simulink model "Main_C0_C3"  (R2023a)
settings: Solver=ode15s  StartTime=0.0  StopTime=1  RelTol=1e-3
model workspace (MAT data in the model file):
  C_IVD = 0.05
  E_IVD1 = 2.1
  E_IVD2 = 2.2
  E_IVD3 = 1.1
  E_IVD4 = 1.7
  E_IVD5 = 3.2
  IVD1 : object (value not decoded)
  IVD2 : object (value not decoded)
  IVD3 : object (value not decoded)
  IVD4 : object (value not decoded)
  IVD5 : object (value not decoded)
  eo_color = [1 0 0]
  io_color = [0 1 0]
  longissimus_color = [1 0 1]
  multifidus_color = [0 1 1]
  muscle_radius = 1
  psoas_color = [0 0 1]
  ra_color = [1 1 0.5]
symbols that are objects in the model workspace (value not decoded): IVD1, IVD2, IVD3, IVD4, IVD5
undefined symbols (not defined in the file or in its folder): AbdFlex, E_TLFflex, IAP_activation_AbdFlex, IAP_Pa, LeftAbdominalMuscleForce, LeftBackMuscleForce, LeftTransverse1MuscleForce, LeftTransverse2MuscleForce, RightAbdominalMuscleForce, RightBackMuscleForce, RightTransverse1MuscleForce, RightTransverse2MuscleForce, TLFflex2, X, Y, Z
libraries: nesl_utility x1235, sm_lib x960, fl_lib x6, simulink_extras x2
(part 12 of 37)

== system Main_C0_C3/Left and Right Intertransverse Ligaments/ITL Visualization - debug/Ligament9 ==
  Constant : Constant  Value=0
  Constant1 : Constant  Value=0
  Gimbal Joint : sm_lib/Joints/Gimbal Joint  JointMode=Normal  SenseConstraintForce=off  SenseConstraintForceX=off  SenseConstraintForceY=off  SenseConstraintForceZ=off  SenseConstraintTorque=off  SenseConstraintTorqueX=off  SenseConstraintTorqueY=off  SenseConstraintTorqueZ=off  SenseTotalForce=off  SenseTotalForceX=off  SenseTotalForceY=off  SenseTotalForceZ=off  SenseTotalTorque=off  SenseTotalTorqueX=off  SenseTotalTorqueY=off  SenseTotalTorqueZ=off  CompositeWrenchDir=FollowerOnBase  CompositeWrenchFrame=BaseFrame  RxEquilibriumPosition=0  RxEquilibriumPositionUnits=deg  RxSpringStiffness=0  RxSpringStiffnessUnits=N*m/deg  RxDampingCoefficient=0  RxDampingCoefficientUnits=N*m/(deg/s)  RxTorqueActuationMode=ComputedTorque  RxMotionActuationMode=InputMotion  RxSensePosition=off  RxSenseVelocity=off  RxSenseAcceleration=off  RxSenseTorqueForce=off  RxSenseLowerLimitTorqueForce=off  RxSenseUpperLimitTorqueForce=off  RxLowerLimitSpecify=off  RxLowerLimitBound=-90  RxLowerLimitBoundUnits=deg  RxLowerLimitStiffness=1e4  RxLowerLimitStiffnessUnits=N*m/deg  RxLowerLimitDamping=10  RxLowerLimitDampingUnits=N*m/(deg/s)  RxLowerLimitTransitionRegionWidth=0.1  RxLowerLimitTransitionRegionWidthUnits=deg  RxUpperLimitSpecify=off  RxUpperLimitBound=90  RxUpperLimitBoundUnits=deg  RxUpperLimitStiffness=1e4  RxUpperLimitStiffnessUnits=N*m/deg  RxUpperLimitDamping=10  RxUpperLimitDampingUnits=N*m/(deg/s)  RxUpperLimitTransitionRegionWidth=0.1  RxUpperLimitTransitionRegionWidthUnits=deg  RxPositionTargetSpecify=off  RxPositionTargetPriority=High  RxPositionTargetValue=0  RxPositionTargetValueUnits=deg  RxVelocityTargetSpecify=off  RxVelocityTargetPriority=High  RxVelocityTargetValue=0  RxVelocityTargetValueUnits=deg/s  RyEquilibriumPosition=0  RyEquilibriumPositionUnits=deg  RySpringStiffness=0  RySpringStiffnessUnits=N*m/deg  RyDampingCoefficient=0  RyDampingCoefficientUnits=N*m/(deg/s)  RyTorqueActuationMode=ComputedTorque  RyMotionActuationMode=InputMotion  RySensePosition=off  RySenseVelocity=off  RySenseAcceleration=off  RySenseTorqueForce=off  RySenseLowerLimitTorqueForce=off  RySenseUpperLimitTorqueForce=off  RyLowerLimitSpecify=off  RyLowerLimitBound=-90  RyLowerLimitBoundUnits=deg  RyLowerLimitStiffness=1e4  RyLowerLimitStiffnessUnits=N*m/deg  RyLowerLimitDamping=10  RyLowerLimitDampingUnits=N*m/(deg/s)  RyLowerLimitTransitionRegionWidth=0.1  RyLowerLimitTransitionRegionWidthUnits=deg  RyUpperLimitSpecify=off  RyUpperLimitBound=90  RyUpperLimitBoundUnits=deg  RyUpperLimitStiffness=1e4  RyUpperLimitStiffnessUnits=N*m/deg  RyUpperLimitDamping=10  RyUpperLimitDampingUnits=N*m/(deg/s)  RyUpperLimitTransitionRegionWidth=0.1  RyUpperLimitTransitionRegionWidthUnits=deg  RyPositionTargetSpecify=off  RyPositionTargetPriority=High  RyPositionTargetValue=0  RyPositionTargetValueUnits=deg  RyVelocityTargetSpecify=off  RyVelocityTargetPriority=High  RyVelocityTargetValue=0  RyVelocityTargetValueUnits=deg/s  RzEquilibriumPosition=0  RzEquilibriumPositionUnits=deg  RzSpringStiffness=0  RzSpringStiffnessUnits=N*m/deg  RzDampingCoefficient=0  RzDampingCoefficientUnits=N*m/(deg/s)  RzTorqueActuationMode=ComputedTorque  RzMotionActuationMode=InputMotion  RzSensePosition=off  RzSenseVelocity=off  RzSenseAcceleration=off  RzSenseTorqueForce=off  RzSenseLowerLimitTorqueForce=off  RzSenseUpperLimitTorqueForce=off  RzLowerLimitSpecify=off  RzLowerLimitBound=-90  RzLowerLimitBoundUnits=deg  RzLowerLimitStiffness=1e4  RzLowerLimitStiffnessUnits=N*m/deg  RzLowerLimitDamping=10  RzLowerLimitDampingUnits=N*m/(deg/s)  RzLowerLimitTransitionRegionWidth=0.1  RzLowerLimitTransitionRegionWidthUnits=deg  RzUpperLimitSpecify=off  RzUpperLimitBound=90  RzUpperLimitBoundUnits=deg  RzUpperLimitStiffness=1e4  RzUpperLimitStiffnessUnits=N*m/deg  RzUpperLimitDamping=10  RzUpperLimitDampingUnits=N*m/(deg/s)  RzUpperLimitTransitionRegionWidth=0.1  RzUpperLimitTransitionRegionWidthUnits=deg  RzPositionTargetSpecify=off  RzPositionTargetPriority=High  RzPositionTargetValue=0  RzPositionTargetValueUnits=deg  RzVelocityTargetSpecify=off  RzVelocityTargetPriority=High  RzVelocityTargetValue=0  RzVelocityTargetValueUnits=deg/s
  MATLAB Function2 : MATLAB Function  TreatAsAtomicUnit=on
  PS-Simulink Converter{,6..7,11..13} (6 alike) : nesl_utility/PS-Simulink Converter  PhysicalDomain=network_engine_domain  SubClassName=ps_output  LeftPortType=input  RightPortType=output  PseudoPeriodic=off  Frequencies=[]  VectorFormat=inherit  Unit=inherit  AffineConversion=off
  Simulink-PS Converter : nesl_utility/Simulink-PS Converter  PhysicalDomain=network_engine_domain  SubClassName=ps_input  LeftPortType=input  RightPortType=output  PseudoPeriodic=off  Frequencies=[]  NoiseDistribution=none  NoiseParameters=[]  Unit=m  AffineConversion=off  FilteringAndDerivatives=provide  SimscapeFilterOrder=1  InputFilterTimeConstant=0.001  UdotUserProvided=0
  Simulink-PS Converter10 : nesl_utility/Simulink-PS Converter  PhysicalDomain=network_engine_domain  SubClassName=ps_input  LeftPortType=input  RightPortType=output  PseudoPeriodic=off  Frequencies=[]  NoiseDistribution=none  NoiseParameters=[]  Unit=1  AffineConversion=off  FilteringAndDerivatives=provide  SimscapeFilterOrder=2  InputFilterTimeConstant=0.001  UdotUserProvided=2
  Simulink-PS Converter11 : nesl_utility/Simulink-PS Converter  PhysicalDomain=network_engine_domain  SubClassName=ps_input  LeftPortType=input  RightPortType=output  PseudoPeriodic=off  Frequencies=[]  NoiseDistribution=none  NoiseParameters=[]  Unit=1  AffineConversion=off  FilteringAndDerivatives=provide  SimscapeFilterOrder=2  InputFilterTimeConstant=0.001  UdotUserProvided=2
  Simulink-PS Converter9 : nesl_utility/Simulink-PS Converter  PhysicalDomain=network_engine_domain  SubClassName=ps_input  LeftPortType=input  RightPortType=output  PseudoPeriodic=off  Frequencies=[]  NoiseDistribution=none  NoiseParameters=[]  Unit=1  AffineConversion=on  FilteringAndDerivatives=provide  SimscapeFilterOrder=2  InputFilterTimeConstant=0.1  UdotUserProvided=2
  Transform Sensor : sm_lib/Frames and Transforms/Transform Sensor  MeasurementFrame=Base  RotationSequence=XYZ  SenseAngle=off  SenseAxis=off  SenseQ=off  SenseR=off  SenseRotationSequence=off  SenseOmegaX=off  SenseOmegaY=off  SenseOmegaZ=off  SenseQDot=off  SenseRDot=off  SenseRotationSequenceDot=off  SenseAlphaX=off  SenseAlphaY=off  SenseAlphaZ=off  SenseQDDot=off  SenseRDDot=off  SenseX=on  SenseY=on  SenseZ=on  SenseRad=off  SenseAzim=off  SenseDist=off  SenseInc=off  SenseXDot=off  SenseYDot=off  SenseZDot=off  SenseRadDot=off  SenseAzimDot=off  SenseDistDot=off  SenseIncDot=off  SenseXDDot=off  SenseYDDot=off  SenseZDDot=off  SenseRadDDot=off  SenseAzimDDot=off  SenseDistDDot=off  SenseIncDDot=off
  Transform Sensor1 : sm_lib/Frames and Transforms/Transform Sensor  MeasurementFrame=Base  RotationSequence=XYZ  SenseAngle=off  SenseAxis=off  SenseQ=off  SenseR=off  SenseRotationSequence=off  SenseOmegaX=off  SenseOmegaY=off  SenseOmegaZ=off  SenseQDot=off  SenseRDot=off  SenseRotationSequenceDot=off  SenseAlphaX=off  SenseAlphaY=off  SenseAlphaZ=off  SenseQDDot=off  SenseRDDot=off  SenseX=on  SenseY=on  SenseZ=on  SenseRad=off  SenseAzim=off  SenseDist=off  SenseInc=off  SenseXDot=off  SenseYDot=off  SenseZDot=off  SenseRadDot=off  SenseAzimDot=off  SenseDistDot=off  SenseIncDot=off  SenseXDDot=off  SenseYDDot=off  SenseZDDot=off  SenseRadDDot=off  SenseAzimDDot=off  SenseDistDDot=off  SenseIncDDot=off
  Transport Delay : TransportDelay  DelayTime=1e-6
  Transport Delay1 : TransportDelay  DelayTime=1e-6
  Transport Delay2 : TransportDelay  DelayTime=1e-6
  Variable Cylindrical Solid : sm_lib/Body Elements/Variable Mass/Variable Cylindrical Solid  LengthType=ProvidedByInput  Length=1  LengthUnits=m  RadiusType=Constant  Radius=ligament_radius  RadiusUnits=mm  MassType=CalculateFromGeometry  InitialMassType=Specified  InitialMass=1  InitialMassUnits=kg  Density=0.1  DensityUnits=kg/m^3  SenseRadius=off  SenseLength=off  SenseMass=off  SenseCenterOfMass=off  SenseInertiaMatrix=off  GraphicType=FromGeometry  MarkerShape=Sphere  MarkerSize=10  GraphicVisPropType=SimpleVisualProperties  GraphicDiffuseColor=ITL_color  GraphicSpecularColor=[0.5 0.5 0.5 1.0]  GraphicAmbientColor=[0.15 0.15 0.15 1.0]  GraphicEmissiveColor=[0.0 0.0 0.0 1.0]  GraphicShininess=75  GraphicOpacity=1.0
  MuscleEnd1 : PMIOPort  Side=Right
  MuscleEnd2 : PMIOPort  Port=2  Side=Right
  R : PMIOPort  Port=3  Side=Right
  wires:
  Constant1/1 -> Simulink-PS Converter9/3, Simulink-PS Converter10/3, Simulink-PS Converter11/3
  Constant/1 -> Simulink-PS Converter9/2, Simulink-PS Converter10/2, Simulink-PS Converter11/2
  MATLAB Function2/1(length) -> Simulink-PS Converter/1
  PS-Simulink Converter6/1 -> MATLAB Function2/2(y1)
  PS-Simulink Converter12/1 -> MATLAB Function2/5(y2)
  Transport Delay2/1 -> Simulink-PS Converter11/1
  MATLAB Function2/2(Rx) -> Transport Delay1/1
  MATLAB Function2/3(Ry) -> Transport Delay/1
  PS-Simulink Converter/1 -> MATLAB Function2/1(x1)
  PS-Simulink Converter13/1 -> MATLAB Function2/6(z2)
  Transport Delay1/1 -> Simulink-PS Converter9/1
  PS-Simulink Converter11/1 -> MATLAB Function2/4(x2)
  MATLAB Function2/4(Rz) -> Transport Delay2/1
  Transport Delay/1 -> Simulink-PS Converter10/1
  PS-Simulink Converter7/1 -> MATLAB Function2/3(z1)
  connections:
  MuscleEnd2/RConn1 -- Transform Sensor1/RConn1
  Simulink-PS Converter/RConn1 -- Variable Cylindrical Solid/LConn1
  Transform Sensor1/RConn3 -- PS-Simulink Converter12/LConn1
  Transform Sensor1/LConn1 -- R/RConn1 -- Transform Sensor/LConn1
  Transform Sensor1/RConn4 -- PS-Simulink Converter13/LConn1
  Transform Sensor/RConn2 -- PS-Simulink Converter/LConn1
  Transform Sensor/RConn3 -- PS-Simulink Converter6/LConn1
  Transform Sensor/RConn1 -- MuscleEnd1/RConn1 -- Gimbal Joint/LConn1
  Transform Sensor1/RConn2 -- PS-Simulink Converter11/LConn1
  Gimbal Joint/RConn1 -- Variable Cylindrical Solid/RConn1
  Simulink-PS Converter11/RConn1 -- Gimbal Joint/LConn4
  Simulink-PS Converter10/RConn1 -- Gimbal Joint/LConn3
  Transform Sensor/RConn4 -- PS-Simulink Converter7/LConn1
  Simulink-PS Converter9/RConn1 -- Gimbal Joint/LConn2

== system Main_C0_C3/Muscle Forces/Muscle Visualization/ExternalOblique Visualization ==
  Muscle49 : Subsystem
  Muscle50 : Subsystem
  Muscle51 : Subsystem
  Muscle52 : Subsystem
  R : PMIOPort  Side=Right
  R1 : PMIOPort  Port=2  Side=Right
  R2 : PMIOPort  Port=3  Side=Right
  R3 : PMIOPort  Port=4  Side=Right
  MuscleEnd2 : PMIOPort  Port=5  Side=Right
  MuscleEnd1 : PMIOPort  Port=6  Side=Right
  MuscleEnd3 : PMIOPort  Port=7  Side=Right
  MuscleEnd4 : PMIOPort  Port=8  Side=Right
  MuscleEnd5 : PMIOPort  Port=9  Side=Right
  MuscleEnd6 : PMIOPort  Port=10  Side=Right
  MuscleEnd7 : PMIOPort  Port=11  Side=Right
  MuscleEnd8 : PMIOPort  Port=12  Side=Right
  connections:
  Muscle50/RConn2 -- MuscleEnd3/RConn1
  Muscle51/RConn2 -- MuscleEnd4/RConn1
  Muscle49/RConn2 -- MuscleEnd2/RConn1
  Muscle49/RConn1 -- MuscleEnd5/RConn1
  Muscle52/RConn2 -- MuscleEnd1/RConn1
  Muscle52/RConn3 -- R3/RConn1
  Muscle50/RConn3 -- R/RConn1
  Muscle51/RConn1 -- MuscleEnd7/RConn1
  Muscle50/RConn1 -- MuscleEnd8/RConn1
  Muscle49/RConn3 -- R2/RConn1
  Muscle51/RConn3 -- R1/RConn1
  Muscle52/RConn1 -- MuscleEnd6/RConn1

== system Main_C0_C3/Muscle Forces/Muscle Visualization/InternalOblique Visualization ==
  Muscle53 : Subsystem
  Muscle54 : Subsystem
  Muscle55 : Subsystem
  Muscle56 : Subsystem
  Muscle57 : Subsystem
  Muscle58 : Subsystem
  R : PMIOPort  Side=Right
  R1 : PMIOPort  Port=2  Side=Right
  R2 : PMIOPort  Port=3  Side=Right
  R3 : PMIOPort  Port=4  Side=Right
  R4 : PMIOPort  Port=5  Side=Right
  R5 : PMIOPort  Port=6  Side=Right
  MuscleEnd2 : PMIOPort  Port=7  Side=Right
  MuscleEnd1 : PMIOPort  Port=8  Side=Right
  MuscleEnd3 : PMIOPort  Port=9  Side=Right
  MuscleEnd4 : PMIOPort  Port=10  Side=Right
  MuscleEnd5 : PMIOPort  Port=11  Side=Right
  MuscleEnd6 : PMIOPort  Port=12  Side=Right
  MuscleEnd7 : PMIOPort  Port=13  Side=Right
  MuscleEnd8 : PMIOPort  Port=14  Side=Right
  MuscleEnd9 : PMIOPort  Port=15  Side=Right
  MuscleEnd10 : PMIOPort  Port=16  Side=Right
  MuscleEnd11 : PMIOPort  Port=17  Side=Right
  MuscleEnd12 : PMIOPort  Port=18  Side=Right
  connections:
  Muscle54/RConn1 -- MuscleEnd8/RConn1
  Muscle56/RConn2 -- MuscleEnd5/RConn1
  Muscle55/RConn3 -- R/RConn1
  Muscle55/RConn2 -- MuscleEnd6/RConn1
  Muscle54/RConn3 -- R2/RConn1
  Muscle58/RConn1 -- MuscleEnd12/RConn1
  Muscle56/RConn1 -- MuscleEnd10/RConn1
  Muscle55/RConn1 -- MuscleEnd9/RConn1
  Muscle53/RConn2 -- MuscleEnd2/RConn1
  Muscle58/RConn3 -- R5/RConn1
  Muscle54/RConn2 -- MuscleEnd3/RConn1
  Muscle57/RConn3 -- R3/RConn1
  Muscle53/RConn1 -- MuscleEnd7/RConn1
  Muscle57/RConn2 -- MuscleEnd4/RConn1
  Muscle57/RConn1 -- MuscleEnd11/RConn1
  Muscle58/RConn2 -- MuscleEnd1/RConn1
  Muscle56/RConn3 -- R1/RConn1
  Muscle53/RConn3 -- R4/RConn1

== system Main_C0_C3/Muscle Forces/Muscle Visualization/Longissimus Visualization ==
  Muscle29 : Subsystem
  Muscle30 : Subsystem
  Muscle31 : Subsystem
  Muscle32 : Subsystem
  Muscle33 : Subsystem
  Muscle34 : Subsystem
  Muscle35 : Subsystem
  Muscle36 : Subsystem
  Muscle37 : Subsystem
  Muscle38 : Subsystem
  Muscle39 : Subsystem
  Muscle40 : Subsystem
  Muscle41 : Subsystem
  Muscle42 : Subsystem
  Muscle43 : Subsystem
  Muscle44 : Subsystem
  Muscle45 : Subsystem
  Muscle46 : Subsystem
  Muscle47 : Subsystem
  Muscle48 : Subsystem
  R : PMIOPort  Side=Left
  MuscleEnd2 : PMIOPort  Port=2  Side=Right
  MuscleEnd1 : PMIOPort  Port=3  Side=Right
  MuscleEnd3 : PMIOPort  Port=4  Side=Left
  MuscleEnd4 : PMIOPort  Port=5  Side=Left
  MuscleEnd5 : PMIOPort  Port=6  Side=Left
  MuscleEnd6 : PMIOPort  Port=7  Side=Right
  MuscleEnd7 : PMIOPort  Port=8  Side=Right
  MuscleEnd8 : PMIOPort  Port=9  Side=Left
  MuscleEnd9 : PMIOPort  Port=10  Side=Right
  MuscleEnd10 : PMIOPort  Port=11  Side=Right
  MuscleEnd11 : PMIOPort  Port=12  Side=Left
  MuscleEnd12 : PMIOPort  Port=13  Side=Right
  MuscleEnd13 : PMIOPort  Port=14  Side=Right
  MuscleEnd14 : PMIOPort  Port=15  Side=Left
  MuscleEnd15 : PMIOPort  Port=16  Side=Right
  MuscleEnd16 : PMIOPort  Port=17  Side=Right
  MuscleEnd17 : PMIOPort  Port=18  Side=Left
  connections:
  Muscle45/RConn2 -- MuscleEnd7/RConn1
  Muscle31/RConn2 -- MuscleEnd9/RConn1
  Muscle48/RConn2 -- MuscleEnd16/RConn1
  Muscle33/RConn2 -- MuscleEnd15/RConn1
  Muscle30/RConn2 -- MuscleEnd6/RConn1
  Muscle29/RConn2 -- MuscleEnd2/RConn1
  Muscle47/RConn2 -- MuscleEnd13/RConn1
  Muscle46/RConn2 -- MuscleEnd10/RConn1
  Muscle32/RConn2 -- MuscleEnd12/RConn1
  Muscle44/RConn2 -- MuscleEnd1/RConn1
  Muscle38/RConn2 -- MuscleEnd17/RConn1 -- Muscle43/RConn2
  Muscle40/RConn2 -- MuscleEnd8/RConn1 -- Muscle35/RConn2
  MuscleEnd14/RConn1 -- Muscle42/RConn2 -- Muscle37/RConn2
  MuscleEnd11/RConn1 -- Muscle41/RConn2 -- Muscle36/RConn2
  Muscle34/RConn2 -- MuscleEnd5/RConn1 -- Muscle39/RConn2
  Muscle32/RConn1 -- Muscle31/RConn1 -- Muscle30/RConn1 -- Muscle34/RConn1 -- Muscle35/RConn1 -- Muscle36/RConn1 -- Muscle37/RConn1 -- Muscle38/RConn1 -- Muscle29/RConn1 -- MuscleEnd3/RConn1 -- Muscle33/RConn1
  Muscle44/RConn1 -- Muscle45/RConn1 -- Muscle46/RConn1 -- Muscle47/RConn1 -- Muscle48/RConn1 -- MuscleEnd4/RConn1 -- Muscle40/RConn1 -- Muscle41/RConn1 -- Muscle42/RConn1 -- Muscle43/RConn1 -- Muscle39/RConn1
  Muscle42/RConn3 -- Muscle41/RConn3 -- Muscle40/RConn3 -- Muscle39/RConn3 -- Muscle34/RConn3 -- Muscle35/RConn3 -- Muscle36/RConn3 -- Muscle37/RConn3 -- Muscle38/RConn3 -- Muscle29/RConn3 -- R/RConn1 -- Muscle30/RConn3 -- Muscle31/RConn3 -- Muscle32/RConn3 -- Muscle33/RConn3 -- Muscle44/RConn3 -- Muscle45/RConn3 -- Muscle46/RConn3 -- Muscle47/RConn3 -- Muscle48/RConn3 -- Muscle43/RConn3

== system Main_C0_C3/Muscle Forces/Muscle Visualization/Multifidus Visualization ==
  Muscle10 : Subsystem
  Muscle11 : Subsystem
  Muscle12 : Subsystem
  Muscle13 : Subsystem
  Muscle14 : Subsystem
  Muscle15 : Subsystem
  Muscle16 : Subsystem
  Muscle17 : Subsystem
  Muscle18 : Subsystem
  Muscle19 : Subsystem
  Muscle20 : Subsystem
  Muscle21 : Subsystem
  Muscle22 : Subsystem
  Muscle23 : Subsystem
  Muscle24 : Subsystem
  Muscle25 : Subsystem
  Muscle26 : Subsystem
  Muscle27 : Subsystem
  Muscle28 : Subsystem
  Muscle9 : Subsystem
  R : PMIOPort  Side=Left
  MuscleEnd2 : PMIOPort  Port=2  Side=Right
  MuscleEnd1 : PMIOPort  Port=3  Side=Right
  MuscleEnd3 : PMIOPort  Port=4  Side=Left
  MuscleEnd4 : PMIOPort  Port=5  Side=Left
  MuscleEnd5 : PMIOPort  Port=6  Side=Right
  MuscleEnd6 : PMIOPort  Port=7  Side=Right
  MuscleEnd7 : PMIOPort  Port=8  Side=Right
  MuscleEnd8 : PMIOPort  Port=9  Side=Right
  MuscleEnd9 : PMIOPort  Port=10  Side=Right
  MuscleEnd10 : PMIOPort  Port=11  Side=Right
  MuscleEnd11 : PMIOPort  Port=12  Side=Right
  MuscleEnd12 : PMIOPort  Port=13  Side=Right
  MuscleEnd13 : PMIOPort  Port=14  Side=Right
  MuscleEnd14 : PMIOPort  Port=15  Side=Left
  MuscleEnd15 : PMIOPort  Port=16  Side=Right
  MuscleEnd16 : PMIOPort  Port=17  Side=Right
  MuscleEnd17 : PMIOPort  Port=18  Side=Left
  connections:
  Muscle9/RConn2 -- MuscleEnd2/RConn1
  Muscle24/RConn2 -- MuscleEnd1/RConn1
  Muscle28/RConn2 -- MuscleEnd15/RConn1
  Muscle25/RConn2 -- MuscleEnd7/RConn1
  Muscle12/RConn2 -- MuscleEnd12/RConn1
  Muscle13/RConn2 -- MuscleEnd16/RConn1
  Muscle16/RConn2 -- MuscleEnd11/RConn1 -- Muscle21/RConn2
  MuscleEnd5/RConn1 -- Muscle19/RConn2 -- Muscle14/RConn2
  Muscle11/RConn2 -- MuscleEnd9/RConn1
  Muscle10/RConn1 -- Muscle11/RConn1 -- Muscle12/RConn1 -- Muscle13/RConn1 -- Muscle14/RConn1 -- Muscle15/RConn1 -- Muscle16/RConn1 -- Muscle17/RConn1 -- Muscle18/RConn1 -- MuscleEnd3/RConn1 -- Muscle9/RConn1
  Muscle25/RConn1 -- Muscle24/RConn1 -- Muscle19/RConn1 -- MuscleEnd4/RConn1 -- Muscle20/RConn1 -- Muscle21/RConn1 -- Muscle22/RConn1 -- Muscle23/RConn1 -- Muscle27/RConn1 -- Muscle28/RConn1 -- Muscle26/RConn1
  Muscle26/RConn2 -- MuscleEnd10/RConn1
  Muscle20/RConn2 -- MuscleEnd8/RConn1 -- Muscle15/RConn2
  Muscle27/RConn2 -- MuscleEnd13/RConn1
  Muscle10/RConn2 -- MuscleEnd6/RConn1
  Muscle10/RConn3 -- Muscle9/RConn3 -- Muscle15/RConn3 -- Muscle16/RConn3 -- Muscle17/RConn3 -- Muscle18/RConn3 -- Muscle14/RConn3 -- Muscle20/RConn3 -- Muscle21/RConn3 -- Muscle23/RConn3 -- Muscle22/RConn3 -- Muscle19/RConn3 -- Muscle24/RConn3 -- Muscle25/RConn3 -- Muscle26/RConn3 -- Muscle27/RConn3 -- Muscle28/RConn3 -- R/RConn1 -- Muscle12/RConn3 -- Muscle13/RConn3 -- Muscle11/RConn3
  Muscle23/RConn2 -- MuscleEnd17/RConn1 -- Muscle18/RConn2
  Muscle17/RConn2 -- MuscleEnd14/RConn1 -- Muscle22/RConn2

== system Main_C0_C3/Muscle Forces/Muscle Visualization/Psoas Visualization ==
  Muscle1 : Subsystem
  Muscle2 : Subsystem
  Muscle3 : Subsystem
  Muscle4 : Subsystem
  Muscle5 : Subsystem
  Muscle6 : Subsystem
  Muscle7 : Subsystem
  Muscle8 : Subsystem
  MuscleEnd2 : PMIOPort  Side=Right
  MuscleEnd1 : PMIOPort  Port=2  Side=Right
  MuscleEnd3 : PMIOPort  Port=3  Side=Left
  MuscleEnd4 : PMIOPort  Port=4  Side=Left
  MuscleEnd5 : PMIOPort  Port=5  Side=Right
  MuscleEnd6 : PMIOPort  Port=6  Side=Right
  MuscleEnd7 : PMIOPort  Port=7  Side=Right
  MuscleEnd8 : PMIOPort  Port=8  Side=Right
  MuscleEnd9 : PMIOPort  Port=9  Side=Right
  MuscleEnd10 : PMIOPort  Port=10  Side=Right
  R : PMIOPort  Port=11  Side=Left
  connections:
  Muscle7/RConn2 -- MuscleEnd7/RConn1
  Muscle6/RConn2 -- MuscleEnd6/RConn1
  Muscle5/RConn2 -- MuscleEnd1/RConn1
  Muscle3/RConn2 -- MuscleEnd8/RConn1
  Muscle2/RConn2 -- MuscleEnd5/RConn1
  Muscle4/RConn1 -- Muscle2/RConn1 -- MuscleEnd3/RConn1 -- Muscle1/RConn1 -- Muscle3/RConn1
  Muscle8/RConn2 -- MuscleEnd9/RConn1
  Muscle7/RConn1 -- Muscle6/RConn1 -- Muscle5/RConn1 -- MuscleEnd4/RConn1 -- Muscle8/RConn1
  Muscle1/RConn2 -- MuscleEnd2/RConn1
  Muscle8/RConn3 -- Muscle7/RConn3 -- Muscle6/RConn3 -- Muscle5/RConn3 -- R/RConn1 -- Muscle3/RConn3 -- Muscle4/RConn3 -- Muscle2/RConn3 -- Muscle1/RConn3
  Muscle4/RConn2 -- MuscleEnd10/RConn1

== system Main_C0_C3/Muscle Forces/Muscle Visualization/RA Visualization ==
  Muscle59 : Subsystem
  Muscle60 : Subsystem
  R : PMIOPort  Side=Left
  MuscleEnd2 : PMIOPort  Port=2  Side=Right
  MuscleEnd1 : PMIOPort  Port=3  Side=Right
  MuscleEnd3 : PMIOPort  Port=4  Side=Right
  MuscleEnd4 : PMIOPort  Port=5  Side=Right
  connections:
  Muscle59/RConn2 -- MuscleEnd1/RConn1
  Muscle60/RConn2 -- MuscleEnd2/RConn1
  Muscle59/RConn1 -- MuscleEnd3/RConn1
  Muscle60/RConn1 -- MuscleEnd4/RConn1
  Muscle60/RConn3 -- R/RConn1 -- Muscle59/RConn3

== system Main_C0_C3/Muscle Forces/Subsystem/Ramped ==
  u : Inport
  Clock : Clock
  MATLAB Function1 : MATLAB Function  TreatAsAtomicUnit=on
  y : Outport
  wires:
  MATLAB Function1/1(y) -> y/1
  Clock/1 -> MATLAB Function1/2(t)
  u/1 -> MATLAB Function1/1(u)

== system Main_C0_C3/Muscle Forces/Subsystem1/Ramped ==
  u : Inport
  Clock : Clock
  MATLAB Function1 : MATLAB Function  TreatAsAtomicUnit=on
  y : Outport
  wires:
  MATLAB Function1/1(y) -> y/1
  Clock/1 -> MATLAB Function1/2(t)
  u/1 -> MATLAB Function1/1(u)

== system Main_C0_C3/Muscle Forces/Subsystem10/Ramped ==
  u : Inport
  Clock : Clock
  MATLAB Function1 : MATLAB Function  TreatAsAtomicUnit=on
  y : Outport
  wires:
  MATLAB Function1/1(y) -> y/1
  Clock/1 -> MATLAB Function1/2(t)
  u/1 -> MATLAB Function1/1(u)

== system Main_C0_C3/Muscle Forces/Subsystem11/Ramped ==
  u : Inport
  Clock : Clock
  MATLAB Function1 : MATLAB Function  TreatAsAtomicUnit=on
  y : Outport
  wires:
  MATLAB Function1/1(y) -> y/1
  Clock/1 -> MATLAB Function1/2(t)
  u/1 -> MATLAB Function1/1(u)

== system Main_C0_C3/Muscle Forces/Subsystem2/Ramped ==
  u : Inport
  Clock : Clock
  MATLAB Function1 : MATLAB Function  TreatAsAtomicUnit=on
  y : Outport
  wires:
  MATLAB Function1/1(y) -> y/1
  Clock/1 -> MATLAB Function1/2(t)
  u/1 -> MATLAB Function1/1(u)

== system Main_C0_C3/Muscle Forces/Subsystem3/Ramped ==
  u : Inport
  Clock : Clock
  MATLAB Function1 : MATLAB Function  TreatAsAtomicUnit=on
  y : Outport
  wires:
  MATLAB Function1/1(y) -> y/1
  Clock/1 -> MATLAB Function1/2(t)
  u/1 -> MATLAB Function1/1(u)

== system Main_C0_C3/Muscle Forces/Subsystem4/Ramped ==
  u : Inport
  Clock : Clock
  MATLAB Function1 : MATLAB Function  TreatAsAtomicUnit=on
  y : Outport
  wires:
  MATLAB Function1/1(y) -> y/1
  Clock/1 -> MATLAB Function1/2(t)
  u/1 -> MATLAB Function1/1(u)

== system Main_C0_C3/Muscle Forces/Subsystem5/Ramped ==
  u : Inport
  Clock : Clock
  MATLAB Function1 : MATLAB Function  TreatAsAtomicUnit=on
  y : Outport
  wires:
  MATLAB Function1/1(y) -> y/1
  Clock/1 -> MATLAB Function1/2(t)
  u/1 -> MATLAB Function1/1(u)

== system Main_C0_C3/Muscle Forces/Subsystem6/Ramped ==
  u : Inport
  Clock : Clock
  MATLAB Function1 : MATLAB Function  TreatAsAtomicUnit=on
  y : Outport
  wires:
  MATLAB Function1/1(y) -> y/1
  Clock/1 -> MATLAB Function1/2(t)
  u/1 -> MATLAB Function1/1(u)

== system Main_C0_C3/Muscle Forces/Subsystem7/Ramped ==
  u : Inport
  Clock : Clock
  MATLAB Function1 : MATLAB Function  TreatAsAtomicUnit=on
  y : Outport
  wires:
  MATLAB Function1/1(y) -> y/1
  Clock/1 -> MATLAB Function1/2(t)
  u/1 -> MATLAB Function1/1(u)

== system Main_C0_C3/Muscle Forces/Subsystem8/Ramped ==
  u : Inport
  Clock : Clock
  MATLAB Function1 : MATLAB Function  TreatAsAtomicUnit=on
  y : Outport
  wires:
  MATLAB Function1/1(y) -> y/1
  Clock/1 -> MATLAB Function1/2(t)
  u/1 -> MATLAB Function1/1(u)

== system Main_C0_C3/Muscle Forces/Subsystem9/Ramped ==
  u : Inport
  Clock : Clock
  MATLAB Function1 : MATLAB Function  TreatAsAtomicUnit=on
  y : Outport
  wires:
  MATLAB Function1/1(y) -> y/1
  Clock/1 -> MATLAB Function1/2(t)
  u/1 -> MATLAB Function1/1(u)

== system Main_C0_C3/Supraspinous Ligaments/SSL Visualization/Ligament1 ==
  Constant : Constant  Value=0
  Constant1 : Constant  Value=0
  Gimbal Joint : sm_lib/Joints/Gimbal Joint  JointMode=Normal  SenseConstraintForce=off  SenseConstraintForceX=off  SenseConstraintForceY=off  SenseConstraintForceZ=off  SenseConstraintTorque=off  SenseConstraintTorqueX=off  SenseConstraintTorqueY=off  SenseConstraintTorqueZ=off  SenseTotalForce=off  SenseTotalForceX=off  SenseTotalForceY=off  SenseTotalForceZ=off  SenseTotalTorque=off  SenseTotalTorqueX=off  SenseTotalTorqueY=off  SenseTotalTorqueZ=off  CompositeWrenchDir=FollowerOnBase  CompositeWrenchFrame=BaseFrame  RxEquilibriumPosition=0  RxEquilibriumPositionUnits=deg  RxSpringStiffness=0  RxSpringStiffnessUnits=N*m/deg  RxDampingCoefficient=0  RxDampingCoefficientUnits=N*m/(deg/s)  RxTorqueActuationMode=ComputedTorque  RxMotionActuationMode=InputMotion  RxSensePosition=off  RxSenseVelocity=off  RxSenseAcceleration=off  RxSenseTorqueForce=off  RxSenseLowerLimitTorqueForce=off  RxSenseUpperLimitTorqueForce=off  RxLowerLimitSpecify=off  RxLowerLimitBound=-90  RxLowerLimitBoundUnits=deg  RxLowerLimitStiffness=1e4  RxLowerLimitStiffnessUnits=N*m/deg  RxLowerLimitDamping=10  RxLowerLimitDampingUnits=N*m/(deg/s)  RxLowerLimitTransitionRegionWidth=0.1  RxLowerLimitTransitionRegionWidthUnits=deg  RxUpperLimitSpecify=off  RxUpperLimitBound=90  RxUpperLimitBoundUnits=deg  RxUpperLimitStiffness=1e4  RxUpperLimitStiffnessUnits=N*m/deg  RxUpperLimitDamping=10  RxUpperLimitDampingUnits=N*m/(deg/s)  RxUpperLimitTransitionRegionWidth=0.1  RxUpperLimitTransitionRegionWidthUnits=deg  RxPositionTargetSpecify=off  RxPositionTargetPriority=High  RxPositionTargetValue=0  RxPositionTargetValueUnits=deg  RxVelocityTargetSpecify=off  RxVelocityTargetPriority=High  RxVelocityTargetValue=0  RxVelocityTargetValueUnits=deg/s  RyEquilibriumPosition=0  RyEquilibriumPositionUnits=deg  RySpringStiffness=0  RySpringStiffnessUnits=N*m/deg  RyDampingCoefficient=0  RyDampingCoefficientUnits=N*m/(deg/s)  RyTorqueActuationMode=ComputedTorque  RyMotionActuationMode=InputMotion  RySensePosition=off  RySenseVelocity=off  RySenseAcceleration=off  RySenseTorqueForce=off  RySenseLowerLimitTorqueForce=off  RySenseUpperLimitTorqueForce=off  RyLowerLimitSpecify=off  RyLowerLimitBound=-90  RyLowerLimitBoundUnits=deg  RyLowerLimitStiffness=1e4  RyLowerLimitStiffnessUnits=N*m/deg  RyLowerLimitDamping=10  RyLowerLimitDampingUnits=N*m/(deg/s)  RyLowerLimitTransitionRegionWidth=0.1  RyLowerLimitTransitionRegionWidthUnits=deg  RyUpperLimitSpecify=off  RyUpperLimitBound=90  RyUpperLimitBoundUnits=deg  RyUpperLimitStiffness=1e4  RyUpperLimitStiffnessUnits=N*m/deg  RyUpperLimitDamping=10  RyUpperLimitDampingUnits=N*m/(deg/s)  RyUpperLimitTransitionRegionWidth=0.1  RyUpperLimitTransitionRegionWidthUnits=deg  RyPositionTargetSpecify=off  RyPositionTargetPriority=High  RyPositionTargetValue=0  RyPositionTargetValueUnits=deg  RyVelocityTargetSpecify=off  RyVelocityTargetPriority=High  RyVelocityTargetValue=0  RyVelocityTargetValueUnits=deg/s  RzEquilibriumPosition=0  RzEquilibriumPositionUnits=deg  RzSpringStiffness=0  RzSpringStiffnessUnits=N*m/deg  RzDampingCoefficient=0  RzDampingCoefficientUnits=N*m/(deg/s)  RzTorqueActuationMode=ComputedTorque  RzMotionActuationMode=InputMotion  RzSensePosition=off  RzSenseVelocity=off  RzSenseAcceleration=off  RzSenseTorqueForce=off  RzSenseLowerLimitTorqueForce=off  RzSenseUpperLimitTorqueForce=off  RzLowerLimitSpecify=off  RzLowerLimitBound=-90  RzLowerLimitBoundUnits=deg  RzLowerLimitStiffness=1e4  RzLowerLimitStiffnessUnits=N*m/deg  RzLowerLimitDamping=10  RzLowerLimitDampingUnits=N*m/(deg/s)  RzLowerLimitTransitionRegionWidth=0.1  RzLowerLimitTransitionRegionWidthUnits=deg  RzUpperLimitSpecify=off  RzUpperLimitBound=90  RzUpperLimitBoundUnits=deg  RzUpperLimitStiffness=1e4  RzUpperLimitStiffnessUnits=N*m/deg  RzUpperLimitDamping=10  RzUpperLimitDampingUnits=N*m/(deg/s)  RzUpperLimitTransitionRegionWidth=0.1  RzUpperLimitTransitionRegionWidthUnits=deg  RzPositionTargetSpecify=off  RzPositionTargetPriority=High  RzPositionTargetValue=0  RzPositionTargetValueUnits=deg  RzVelocityTargetSpecify=off  RzVelocityTargetPriority=High  RzVelocityTargetValue=0  RzVelocityTargetValueUnits=deg/s
  MATLAB Function2 : MATLAB Function  TreatAsAtomicUnit=on
  PS-Simulink Converter{,6..7,11..13} (6 alike) : nesl_utility/PS-Simulink Converter  PhysicalDomain=network_engine_domain  SubClassName=ps_output  LeftPortType=input  RightPortType=output  PseudoPeriodic=off  Frequencies=[]  VectorFormat=inherit  Unit=inherit  AffineConversion=off
  Simulink-PS Converter : nesl_utility/Simulink-PS Converter  PhysicalDomain=network_engine_domain  SubClassName=ps_input  LeftPortType=input  RightPortType=output  PseudoPeriodic=off  Frequencies=[]  NoiseDistribution=none  NoiseParameters=[]  Unit=m  AffineConversion=off  FilteringAndDerivatives=provide  SimscapeFilterOrder=1  InputFilterTimeConstant=0.001  UdotUserProvided=0
  Simulink-PS Converter10 : nesl_utility/Simulink-PS Converter  PhysicalDomain=network_engine_domain  SubClassName=ps_input  LeftPortType=input  RightPortType=output  PseudoPeriodic=off  Frequencies=[]  NoiseDistribution=none  NoiseParameters=[]  Unit=1  AffineConversion=off  FilteringAndDerivatives=provide  SimscapeFilterOrder=2  InputFilterTimeConstant=0.001  UdotUserProvided=2
  Simulink-PS Converter11 : nesl_utility/Simulink-PS Converter  PhysicalDomain=network_engine_domain  SubClassName=ps_input  LeftPortType=input  RightPortType=output  PseudoPeriodic=off  Frequencies=[]  NoiseDistribution=none  NoiseParameters=[]  Unit=1  AffineConversion=off  FilteringAndDerivatives=provide  SimscapeFilterOrder=2  InputFilterTimeConstant=0.001  UdotUserProvided=2
  Simulink-PS Converter9 : nesl_utility/Simulink-PS Converter  PhysicalDomain=network_engine_domain  SubClassName=ps_input  LeftPortType=input  RightPortType=output  PseudoPeriodic=off  Frequencies=[]  NoiseDistribution=none  NoiseParameters=[]  Unit=1  AffineConversion=on  FilteringAndDerivatives=provide  SimscapeFilterOrder=2  InputFilterTimeConstant=0.1  UdotUserProvided=2
  Transform Sensor : sm_lib/Frames and Transforms/Transform Sensor  MeasurementFrame=Base  RotationSequence=XYZ  SenseAngle=off  SenseAxis=off  SenseQ=off  SenseR=off  SenseRotationSequence=off  SenseOmegaX=off  SenseOmegaY=off  SenseOmegaZ=off  SenseQDot=off  SenseRDot=off  SenseRotationSequenceDot=off  SenseAlphaX=off  SenseAlphaY=off  SenseAlphaZ=off  SenseQDDot=off  SenseRDDot=off  SenseX=on  SenseY=on  SenseZ=on  SenseRad=off  SenseAzim=off  SenseDist=off  SenseInc=off  SenseXDot=off  SenseYDot=off  SenseZDot=off  SenseRadDot=off  SenseAzimDot=off  SenseDistDot=off  SenseIncDot=off  SenseXDDot=off  SenseYDDot=off  SenseZDDot=off  SenseRadDDot=off  SenseAzimDDot=off  SenseDistDDot=off  SenseIncDDot=off
  Transform Sensor1 : sm_lib/Frames and Transforms/Transform Sensor  MeasurementFrame=Base  RotationSequence=XYZ  SenseAngle=off  SenseAxis=off  SenseQ=off  SenseR=off  SenseRotationSequence=off  SenseOmegaX=off  SenseOmegaY=off  SenseOmegaZ=off  SenseQDot=off  SenseRDot=off  SenseRotationSequenceDot=off  SenseAlphaX=off  SenseAlphaY=off  SenseAlphaZ=off  SenseQDDot=off  SenseRDDot=off  SenseX=on  SenseY=on  SenseZ=on  SenseRad=off  SenseAzim=off  SenseDist=off  SenseInc=off  SenseXDot=off  SenseYDot=off  SenseZDot=off  SenseRadDot=off  SenseAzimDot=off  SenseDistDot=off  SenseIncDot=off  SenseXDDot=off  SenseYDDot=off  SenseZDDot=off  SenseRadDDot=off  SenseAzimDDot=off  SenseDistDDot=off  SenseIncDDot=off
  Transport Delay : TransportDelay  DelayTime=1e-6
  Transport Delay1 : TransportDelay  DelayTime=1e-6
  Transport Delay2 : TransportDelay  DelayTime=1e-6
  Variable Cylindrical Solid : sm_lib/Body Elements/Variable Mass/Variable Cylindrical Solid  LengthType=ProvidedByInput  Length=1  LengthUnits=m  RadiusType=Constant  Radius=ligament_radius  RadiusUnits=mm  MassType=CalculateFromGeometry  InitialMassType=Specified  InitialMass=1  InitialMassUnits=kg  Density=0.1  DensityUnits=kg/m^3  SenseRadius=off  SenseLength=off  SenseMass=off  SenseCenterOfMass=off  SenseInertiaMatrix=off  GraphicType=FromGeometry  MarkerShape=Sphere  MarkerSize=10  GraphicVisPropType=SimpleVisualProperties  GraphicDiffuseColor=SSL_color  GraphicSpecularColor=[0.5 0.5 0.5 1.0]  GraphicAmbientColor=[0.15 0.15 0.15 1.0]  GraphicEmissiveColor=[0.0 0.0 0.0 1.0]  GraphicShininess=75  GraphicOpacity=1.0
  MuscleEnd1 : PMIOPort  Side=Right
  MuscleEnd2 : PMIOPort  Port=2  Side=Right
  R : PMIOPort  Port=3  Side=Right
  wires:
  Constant1/1 -> Simulink-PS Converter9/3, Simulink-PS Converter10/3, Simulink-PS Converter11/3
  Constant/1 -> Simulink-PS Converter9/2, Simulink-PS Converter10/2, Simulink-PS Converter11/2
  MATLAB Function2/1(length) -> Simulink-PS Converter/1
  PS-Simulink Converter6/1 -> MATLAB Function2/2(y1)
  PS-Simulink Converter12/1 -> MATLAB Function2/5(y2)
  Transport Delay2/1 -> Simulink-PS Converter11/1
  MATLAB Function2/2(Rx) -> Transport Delay1/1
  MATLAB Function2/3(Ry) -> Transport Delay/1
  PS-Simulink Converter/1 -> MATLAB Function2/1(x1)
  PS-Simulink Converter13/1 -> MATLAB Function2/6(z2)
  Transport Delay1/1 -> Simulink-PS Converter9/1
  PS-Simulink Converter11/1 -> MATLAB Function2/4(x2)
  MATLAB Function2/4(Rz) -> Transport Delay2/1
  Transport Delay/1 -> Simulink-PS Converter10/1
  PS-Simulink Converter7/1 -> MATLAB Function2/3(z1)
  connections:
  MuscleEnd2/RConn1 -- Transform Sensor1/RConn1
  Simulink-PS Converter/RConn1 -- Variable Cylindrical Solid/LConn1
  Transform Sensor1/RConn3 -- PS-Simulink Converter12/LConn1
  Transform Sensor1/LConn1 -- R/RConn1 -- Transform Sensor/LConn1
  Transform Sensor1/RConn4 -- PS-Simulink Converter13/LConn1
  Transform Sensor/RConn2 -- PS-Simulink Converter/LConn1
  Transform Sensor/RConn3 -- PS-Simulink Converter6/LConn1
  Transform Sensor/RConn1 -- MuscleEnd1/RConn1 -- Gimbal Joint/LConn1
  Transform Sensor1/RConn2 -- PS-Simulink Converter11/LConn1
  Gimbal Joint/RConn1 -- Variable Cylindrical Solid/RConn1
  Simulink-PS Converter11/RConn1 -- Gimbal Joint/LConn4
  Simulink-PS Converter10/RConn1 -- Gimbal Joint/LConn3
  Transform Sensor/RConn4 -- PS-Simulink Converter7/LConn1
  Simulink-PS Converter9/RConn1 -- Gimbal Joint/LConn2

== system Main_C0_C3/Supraspinous Ligaments/SSL Visualization/Ligament2 ==
  Constant : Constant  Value=0
  Constant1 : Constant  Value=0
  Gimbal Joint : sm_lib/Joints/Gimbal Joint  JointMode=Normal  SenseConstraintForce=off  SenseConstraintForceX=off  SenseConstraintForceY=off  SenseConstraintForceZ=off  SenseConstraintTorque=off  SenseConstraintTorqueX=off  SenseConstraintTorqueY=off  SenseConstraintTorqueZ=off  SenseTotalForce=off  SenseTotalForceX=off  SenseTotalForceY=off  SenseTotalForceZ=off  SenseTotalTorque=off  SenseTotalTorqueX=off  SenseTotalTorqueY=off  SenseTotalTorqueZ=off  CompositeWrenchDir=FollowerOnBase  CompositeWrenchFrame=BaseFrame  RxEquilibriumPosition=0  RxEquilibriumPositionUnits=deg  RxSpringStiffness=0  RxSpringStiffnessUnits=N*m/deg  RxDampingCoefficient=0  RxDampingCoefficientUnits=N*m/(deg/s)  RxTorqueActuationMode=ComputedTorque  RxMotionActuationMode=InputMotion  RxSensePosition=off  RxSenseVelocity=off  RxSenseAcceleration=off  RxSenseTorqueForce=off  RxSenseLowerLimitTorqueForce=off  RxSenseUpperLimitTorqueForce=off  RxLowerLimitSpecify=off  RxLowerLimitBound=-90  RxLowerLimitBoundUnits=deg  RxLowerLimitStiffness=1e4  RxLowerLimitStiffnessUnits=N*m/deg  RxLowerLimitDamping=10  RxLowerLimitDampingUnits=N*m/(deg/s)  RxLowerLimitTransitionRegionWidth=0.1  RxLowerLimitTransitionRegionWidthUnits=deg  RxUpperLimitSpecify=off  RxUpperLimitBound=90  RxUpperLimitBoundUnits=deg  RxUpperLimitStiffness=1e4  RxUpperLimitStiffnessUnits=N*m/deg  RxUpperLimitDamping=10  RxUpperLimitDampingUnits=N*m/(deg/s)  RxUpperLimitTransitionRegionWidth=0.1  RxUpperLimitTransitionRegionWidthUnits=deg  RxPositionTargetSpecify=off  RxPositionTargetPriority=High  RxPositionTargetValue=0  RxPositionTargetValueUnits=deg  RxVelocityTargetSpecify=off  RxVelocityTargetPriority=High  RxVelocityTargetValue=0  RxVelocityTargetValueUnits=deg/s  RyEquilibriumPosition=0  RyEquilibriumPositionUnits=deg  RySpringStiffness=0  RySpringStiffnessUnits=N*m/deg  RyDampingCoefficient=0  RyDampingCoefficientUnits=N*m/(deg/s)  RyTorqueActuationMode=ComputedTorque  RyMotionActuationMode=InputMotion  RySensePosition=off  RySenseVelocity=off  RySenseAcceleration=off  RySenseTorqueForce=off  RySenseLowerLimitTorqueForce=off  RySenseUpperLimitTorqueForce=off  RyLowerLimitSpecify=off  RyLowerLimitBound=-90  RyLowerLimitBoundUnits=deg  RyLowerLimitStiffness=1e4  RyLowerLimitStiffnessUnits=N*m/deg  RyLowerLimitDamping=10  RyLowerLimitDampingUnits=N*m/(deg/s)  RyLowerLimitTransitionRegionWidth=0.1  RyLowerLimitTransitionRegionWidthUnits=deg  RyUpperLimitSpecify=off  RyUpperLimitBound=90  RyUpperLimitBoundUnits=deg  RyUpperLimitStiffness=1e4  RyUpperLimitStiffnessUnits=N*m/deg  RyUpperLimitDamping=10  RyUpperLimitDampingUnits=N*m/(deg/s)  RyUpperLimitTransitionRegionWidth=0.1  RyUpperLimitTransitionRegionWidthUnits=deg  RyPositionTargetSpecify=off  RyPositionTargetPriority=High  RyPositionTargetValue=0  RyPositionTargetValueUnits=deg  RyVelocityTargetSpecify=off  RyVelocityTargetPriority=High  RyVelocityTargetValue=0  RyVelocityTargetValueUnits=deg/s  RzEquilibriumPosition=0  RzEquilibriumPositionUnits=deg  RzSpringStiffness=0  RzSpringStiffnessUnits=N*m/deg  RzDampingCoefficient=0  RzDampingCoefficientUnits=N*m/(deg/s)  RzTorqueActuationMode=ComputedTorque  RzMotionActuationMode=InputMotion  RzSensePosition=off  RzSenseVelocity=off  RzSenseAcceleration=off  RzSenseTorqueForce=off  RzSenseLowerLimitTorqueForce=off  RzSenseUpperLimitTorqueForce=off  RzLowerLimitSpecify=off  RzLowerLimitBound=-90  RzLowerLimitBoundUnits=deg  RzLowerLimitStiffness=1e4  RzLowerLimitStiffnessUnits=N*m/deg  RzLowerLimitDamping=10  RzLowerLimitDampingUnits=N*m/(deg/s)  RzLowerLimitTransitionRegionWidth=0.1  RzLowerLimitTransitionRegionWidthUnits=deg  RzUpperLimitSpecify=off  RzUpperLimitBound=90  RzUpperLimitBoundUnits=deg  RzUpperLimitStiffness=1e4  RzUpperLimitStiffnessUnits=N*m/deg  RzUpperLimitDamping=10  RzUpperLimitDampingUnits=N*m/(deg/s)  RzUpperLimitTransitionRegionWidth=0.1  RzUpperLimitTransitionRegionWidthUnits=deg  RzPositionTargetSpecify=off  RzPositionTargetPriority=High  RzPositionTargetValue=0  RzPositionTargetValueUnits=deg  RzVelocityTargetSpecify=off  RzVelocityTargetPriority=High  RzVelocityTargetValue=0  RzVelocityTargetValueUnits=deg/s
  MATLAB Function2 : MATLAB Function  TreatAsAtomicUnit=on
  PS-Simulink Converter{,6..7,11..13} (6 alike) : nesl_utility/PS-Simulink Converter  PhysicalDomain=network_engine_domain  SubClassName=ps_output  LeftPortType=input  RightPortType=output  PseudoPeriodic=off  Frequencies=[]  VectorFormat=inherit  Unit=inherit  AffineConversion=off
  Simulink-PS Converter : nesl_utility/Simulink-PS Converter  PhysicalDomain=network_engine_domain  SubClassName=ps_input  LeftPortType=input  RightPortType=output  PseudoPeriodic=off  Frequencies=[]  NoiseDistribution=none  NoiseParameters=[]  Unit=m  AffineConversion=off  FilteringAndDerivatives=provide  SimscapeFilterOrder=1  InputFilterTimeConstant=0.001  UdotUserProvided=0
  Simulink-PS Converter10 : nesl_utility/Simulink-PS Converter  PhysicalDomain=network_engine_domain  SubClassName=ps_input  LeftPortType=input  RightPortType=output  PseudoPeriodic=off  Frequencies=[]  NoiseDistribution=none  NoiseParameters=[]  Unit=1  AffineConversion=off  FilteringAndDerivatives=provide  SimscapeFilterOrder=2  InputFilterTimeConstant=0.001  UdotUserProvided=2
  Simulink-PS Converter11 : nesl_utility/Simulink-PS Converter  PhysicalDomain=network_engine_domain  SubClassName=ps_input  LeftPortType=input  RightPortType=output  PseudoPeriodic=off  Frequencies=[]  NoiseDistribution=none  NoiseParameters=[]  Unit=1  AffineConversion=off  FilteringAndDerivatives=provide  SimscapeFilterOrder=2  InputFilterTimeConstant=0.001  UdotUserProvided=2
  Simulink-PS Converter9 : nesl_utility/Simulink-PS Converter  PhysicalDomain=network_engine_domain  SubClassName=ps_input  LeftPortType=input  RightPortType=output  PseudoPeriodic=off  Frequencies=[]  NoiseDistribution=none  NoiseParameters=[]  Unit=1  AffineConversion=on  FilteringAndDerivatives=provide  SimscapeFilterOrder=2  InputFilterTimeConstant=0.1  UdotUserProvided=2
  Transform Sensor : sm_lib/Frames and Transforms/Transform Sensor  MeasurementFrame=Base  RotationSequence=XYZ  SenseAngle=off  SenseAxis=off  SenseQ=off  SenseR=off  SenseRotationSequence=off  SenseOmegaX=off  SenseOmegaY=off  SenseOmegaZ=off  SenseQDot=off  SenseRDot=off  SenseRotationSequenceDot=off  SenseAlphaX=off  SenseAlphaY=off  SenseAlphaZ=off  SenseQDDot=off  SenseRDDot=off  SenseX=on  SenseY=on  SenseZ=on  SenseRad=off  SenseAzim=off  SenseDist=off  SenseInc=off  SenseXDot=off  SenseYDot=off  SenseZDot=off  SenseRadDot=off  SenseAzimDot=off  SenseDistDot=off  SenseIncDot=off  SenseXDDot=off  SenseYDDot=off  SenseZDDot=off  SenseRadDDot=off  SenseAzimDDot=off  SenseDistDDot=off  SenseIncDDot=off
  Transform Sensor1 : sm_lib/Frames and Transforms/Transform Sensor  MeasurementFrame=Base  RotationSequence=XYZ  SenseAngle=off  SenseAxis=off  SenseQ=off  SenseR=off  SenseRotationSequence=off  SenseOmegaX=off  SenseOmegaY=off  SenseOmegaZ=off  SenseQDot=off  SenseRDot=off  SenseRotationSequenceDot=off  SenseAlphaX=off  SenseAlphaY=off  SenseAlphaZ=off  SenseQDDot=off  SenseRDDot=off  SenseX=on  SenseY=on  SenseZ=on  SenseRad=off  SenseAzim=off  SenseDist=off  SenseInc=off  SenseXDot=off  SenseYDot=off  SenseZDot=off  SenseRadDot=off  SenseAzimDot=off  SenseDistDot=off  SenseIncDot=off  SenseXDDot=off  SenseYDDot=off  SenseZDDot=off  SenseRadDDot=off  SenseAzimDDot=off  SenseDistDDot=off  SenseIncDDot=off
  Transport Delay : TransportDelay  DelayTime=1e-6
  Transport Delay1 : TransportDelay  DelayTime=1e-6
  Transport Delay2 : TransportDelay  DelayTime=1e-6
  Variable Cylindrical Solid : sm_lib/Body Elements/Variable Mass/Variable Cylindrical Solid  LengthType=ProvidedByInput  Length=1  LengthUnits=m  RadiusType=Constant  Radius=ligament_radius  RadiusUnits=mm  MassType=CalculateFromGeometry  InitialMassType=Specified  InitialMass=1  InitialMassUnits=kg  Density=0.1  DensityUnits=kg/m^3  SenseRadius=off  SenseLength=off  SenseMass=off  SenseCenterOfMass=off  SenseInertiaMatrix=off  GraphicType=FromGeometry  MarkerShape=Sphere  MarkerSize=10  GraphicVisPropType=SimpleVisualProperties  GraphicDiffuseColor=SSL_color  GraphicSpecularColor=[0.5 0.5 0.5 1.0]  GraphicAmbientColor=[0.15 0.15 0.15 1.0]  GraphicEmissiveColor=[0.0 0.0 0.0 1.0]  GraphicShininess=75  GraphicOpacity=1.0
  MuscleEnd1 : PMIOPort  Side=Right
  MuscleEnd2 : PMIOPort  Port=2  Side=Right
  R : PMIOPort  Port=3  Side=Right
  wires:
  Constant1/1 -> Simulink-PS Converter9/3, Simulink-PS Converter10/3, Simulink-PS Converter11/3
  Constant/1 -> Simulink-PS Converter9/2, Simulink-PS Converter10/2, Simulink-PS Converter11/2
  MATLAB Function2/1(length) -> Simulink-PS Converter/1
  PS-Simulink Converter6/1 -> MATLAB Function2/2(y1)
  PS-Simulink Converter12/1 -> MATLAB Function2/5(y2)
  Transport Delay2/1 -> Simulink-PS Converter11/1
  MATLAB Function2/2(Rx) -> Transport Delay1/1
  MATLAB Function2/3(Ry) -> Transport Delay/1
  PS-Simulink Converter/1 -> MATLAB Function2/1(x1)
  PS-Simulink Converter13/1 -> MATLAB Function2/6(z2)
  Transport Delay1/1 -> Simulink-PS Converter9/1
  PS-Simulink Converter11/1 -> MATLAB Function2/4(x2)
  MATLAB Function2/4(Rz) -> Transport Delay2/1
  Transport Delay/1 -> Simulink-PS Converter10/1
  PS-Simulink Converter7/1 -> MATLAB Function2/3(z1)
  connections:
  MuscleEnd2/RConn1 -- Transform Sensor1/RConn1
  Simulink-PS Converter/RConn1 -- Variable Cylindrical Solid/LConn1
  Transform Sensor1/RConn3 -- PS-Simulink Converter12/LConn1
  Transform Sensor1/LConn1 -- R/RConn1 -- Transform Sensor/LConn1
  Transform Sensor1/RConn4 -- PS-Simulink Converter13/LConn1
  Transform Sensor/RConn2 -- PS-Simulink Converter/LConn1
  Transform Sensor/RConn3 -- PS-Simulink Converter6/LConn1
  Transform Sensor/RConn1 -- MuscleEnd1/RConn1 -- Gimbal Joint/LConn1
  Transform Sensor1/RConn2 -- PS-Simulink Converter11/LConn1
  Gimbal Joint/RConn1 -- Variable Cylindrical Solid/RConn1
  Simulink-PS Converter11/RConn1 -- Gimbal Joint/LConn4
  Simulink-PS Converter10/RConn1 -- Gimbal Joint/LConn3
  Transform Sensor/RConn4 -- PS-Simulink Converter7/LConn1
  Simulink-PS Converter9/RConn1 -- Gimbal Joint/LConn2
